simulink model "clk_tree_2"  (Simulink 7.0)
settings: Solver=ode45  StartTime=0.0  StopTime=40e-6  MaxStep=0.1e-9  RelTol=1e-3
InitFcn:
  | bit_rate=400e6;
libraries: powerlib x35, simulink x6, dspsigops x4, dspstat3 x2, commrandsrc2 x1, dspbuff3 x1, dspsnks4 x1
settings Model: Creator=dbenson  LastModifiedBy=dbenson
settings OptimizationCC: InlineInvariantSignals=on
settings DebuggingCC: SaveWithParameterizedLinksMsg=none  SignalResolutionControl=TryResolveAllWithWarning  MultiTaskDSMMsg=warning  MultiTaskCondExecSysMsg=none  StrictBusMsg=None
settings RTWCC: IncludeERTFirstTime=on
settings GRTTargetCC: TargetFcnLib=ansi_tfl_tmw.mat

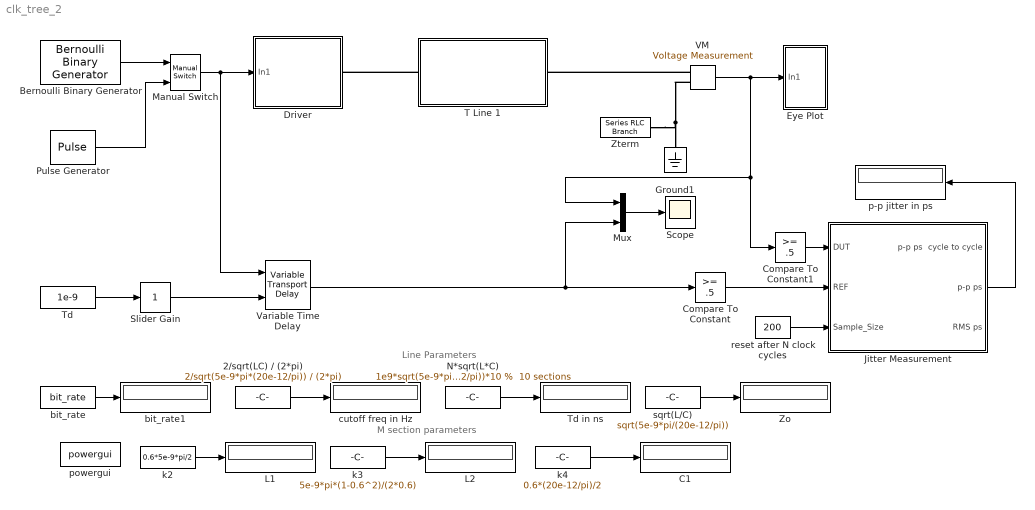
== system clk_tree_2 ==
  note: Line Parameters
  note: M section parameters
  2/sqrt(LC) / (2*pi) : Constant  Value=2/sqrt(5e-9*pi*(20e-12/pi)) / (2*pi)  OutDataType=sfix(16)  OutScaling=2^0
  Bernoulli Binary Generator : commrandsrc2/Bernoulli Binary Generator  DialogController=commDDGCreate  DialogControllerArgs=DataTag0  SystemSampleTime=-1  P=0.5  seed=61  Ts=1/bit_rate  frameBased=off  sampPerFrame=1  orient=off  outDataType=double
  C1 : Display
  Compare To Constant : simulink/Logic and Bit Operations/Compare To Constant  SystemSampleTime=-1  relop=>=  const=.5  LogicOutDataTypeMode=boolean  ZeroCross=off
  Compare To Constant1 : simulink/Logic and Bit Operations/Compare To Constant  SystemSampleTime=-1  relop=>=  const=.5  LogicOutDataTypeMode=boolean  ZeroCross=off
  Driver : Subsystem
  Eye Plot : Subsystem
  Ground1 : powerlib/Elements/Ground  Orientation=down  DialogController=POWERSYS.PowerSysDialog  PhysicalDomain=powersysdomain  SubClassName=unknown  LeftPortType=p1  RightPortType=p1  LConnTagsString=a
  "Jitter Measurement " : Subsystem
  L1 : Display
  L2 : Display
  Manual Switch : simulink/Signal Routing/Manual Switch  SystemSampleTime=-1  sw=1  action=0  varsize=off
  Mux : Mux  Inputs=2
  N*sqrt(L*C) : Constant  Value="1e9*sqrt(5e-9*pi*(20e-12/pi))*10 %  10 sections"  OutDataType=sfix(16)  OutScaling=2^0
  Pulse Generator : DiscretePulseGenerator  PulseType=Time based  Period=2/bit_rate  PulseWidth=50
  Scope : Scope
      settings: TimeRange=1e-008  YMin=-0.4162746057435363  YMax=1.209680454665211
  Slider Gain : simulink/Math Operations/Slider Gain  SystemSampleTime=-1  low=0  gain=1  high=5
  T Line 1 : Subsystem
  Td : Constant  Value=1e-9  OutDataType=sfix(16)  OutScaling=2^0
  Td in ns : Display
  VM : powerlib/Measurements/Voltage Measurement  DialogController=POWERSYS.PowerSysDialog  SystemSampleTime=-1  PhasorSimulation=off  OutputType=Complex  PSBequivalent=0
  Variable Time Delay : VariableTransportDelay  MaximumDelay=10e-9
  Zo : Display
  Zterm : powerlib/Elements/Series RLC Branch  DialogController=POWERSYS.PowerSysDialog  PhysicalDomain=powersysdomain  SubClassName=unknown  LeftPortType=p1  RightPortType=p1  LConnTagsString=__new0  RConnTagsString=__new0  BranchType=R  Resistance=50  Inductance=1e-3  SetiL0=off  InitialCurrent=0  Capacitance=1e-6  Setx0=off  InitialVoltage=0  Measurements=None
  bit_rate : Constant  Value=bit_rate  OutDataType=sfix(16)  OutScaling=2^0
  bit_rate1 : Display
  cutoff freq in Hz : Display
  k2 : Constant  Value=0.6*5e-9*pi/2  OutDataType=sfix(16)  OutScaling=2^0
  k3 : Constant  Value=5e-9*pi*(1-0.6^2)/(2*0.6)  OutDataType=sfix(16)  OutScaling=2^0
  k4 : Constant  Value=0.6*(20e-12/pi)/2  OutDataType=sfix(16)  OutScaling=2^0
  p-p jitter in ps : Display
  powergui : powerlib/powergui  SystemSampleTime=-1  SimulationMode=Continuous  SampleTime=50e-6  echomessages=off  RestoreLinks=warning  x0status=blocks  Frange=[0:2:500]  Ylog=off  Xlog=on  ShowGrid=off  save=off  variable=ZData  ZoomFFT=on  StartTime=0.0  cycles=1  DisplayStyle=1  fundamental=60  FreqAxis=off  MaxFrequency=1000  frequencyindice=0  frequencyindicesteady=1  RmsSteady=1  display=off  Ts=0  frequency=60  methode=off  HookPort=off  Interpol=off  SPID=off  FunctionMessages=off
  reset after N clock cycles : Constant  Value=200  VectorParams1D=off  OutDataType=sfix(16)  OutScaling=2^0
  sqrt(L/C) : Constant  Value=sqrt(5e-9*pi/(20e-12/pi))  OutDataType=sfix(16)  OutScaling=2^0
  wires:
  sqrt(L/C)/1 -> Zo/1
  N*sqrt(L*C)/1 -> Td in ns/1
  k2/1 -> L1/1
  k3/1 -> L2/1
  k4/1 -> C1/1
  2/sqrt(LC) / (2*pi)/1 -> cutoff freq in Hz/1
  VM/1 -> Eye Plot/1(In1), Mux/1, Compare To Constant1/1
  bit_rate/1 -> bit_rate1/1
  Pulse Generator/1 -> Manual Switch/2
  Bernoulli Binary Generator/1 -> Manual Switch/1
  Manual Switch/1 -> Driver/1(In1), Variable Time Delay/1
  "Jitter Measurement "/2(p-p ps) -> p-p jitter in ps/1
  reset after N clock cycles/1 -> "Jitter Measurement "/3(Sample_Size)
  Variable Time Delay/1 -> Mux/2, Compare To Constant/1
  Td/1 -> Slider Gain/1
  Mux/1 -> Scope/1
  Slider Gain/1 -> Variable Time Delay/2
  Compare To Constant/1 -> "Jitter Measurement "/2(REF)
  Compare To Constant1/1 -> "Jitter Measurement "/1(DUT)
  connections:
  T Line 1/LConn1 -- Driver/RConn1
  VM/LConn2 -- Ground1/LConn1 -- Zterm/RConn1
  VM/LConn1 -- T Line 1/RConn1

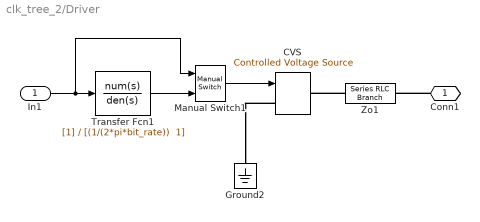
== system clk_tree_2/Driver ==
  In1 : Inport
  CVS : powerlib/Electrical Sources/Controlled Voltage Source  Description=source block  DialogController=POWERSYS.PowerSysDialog  SystemSampleTime=-1  Initialize=off  Source_Type=AC  Amplitude=0  Phase=0  Frequency=0  Measurements=None
      settings: AttributesFormatString=\n
  Ground2 : powerlib/Elements/Ground  Orientation=down  DialogController=POWERSYS.PowerSysDialog  PhysicalDomain=powersysdomain  SubClassName=unknown  LeftPortType=p1  RightPortType=p1  LConnTagsString=a
  Manual Switch1 : simulink/Signal Routing/Manual Switch  SystemSampleTime=-1  sw=0  action=0  varsize=off
  Transfer Fcn1 : TransferFcn  Denominator="[(1/(2*pi*bit_rate))  1]"
  Zo1 : powerlib/Elements/Series RLC Branch  DialogController=POWERSYS.PowerSysDialog  PhysicalDomain=powersysdomain  SubClassName=unknown  LeftPortType=p1  RightPortType=p1  LConnTagsString=__new0  RConnTagsString=__new0  BranchType=R  Resistance=50  Inductance=1e-3  SetiL0=off  InitialCurrent=0  Capacitance=1e-6  Setx0=off  InitialVoltage=0  Measurements=None
  Conn1 : PMIOPort  Orientation=left  Port=1  Side=Right
  wires:
  In1/1 -> Manual Switch1/1, Transfer Fcn1/1
  Manual Switch1/1 -> CVS/1
  Transfer Fcn1/1 -> Manual Switch1/2
  connections:
  CVS/LConn1 -- Ground2/LConn1
  Zo1/LConn1 -- CVS/RConn1
  Conn1/RConn1 -- Zo1/RConn1

== system clk_tree_2/Eye Plot ==
  In1 : Inport
  Buffer : dspbuff3/Buffer  N=200  V=0  ic=0
  Vector Scope1 : dspsnks4/Vector Scope  DialogController=dspdialog.VectorScope  DialogControllerArgs=DataTag1  ScopeProperties=on  Domain=User-defined  HorizSpan=1  DisplayProperties=off  AxisGrid=on  Memory=on  FrameNumber=on  AxisLegend=off  AxisZoom=off  OpenScopeAtSimStart=on  OpenScopeImmediately=off  FigPos=[3 39 417 270]  AxisProperties=off  XUnits=Hertz  XRange=[0...Fs/2]  InheritXIncr=off  XIncr=.01/bit_rate  XLabel=Time  XLimit=Auto  XMin=0  XMax=1  XStart=0  YUnits=dB  YLabel=Amplitude  LineProperties=off  LineColors=[0 0 1]|[1 0 0]
      settings: YMin=-0.298875449569035  YMax=1.30250670189524
  Zero-Order Hold1 : ZeroOrderHold  SampleTime=.01/bit_rate
  wires:
  Zero-Order Hold1/1 -> Buffer/1  "Clock"
  Buffer/1 -> Vector Scope1/1
  In1/1 -> Zero-Order Hold1/1

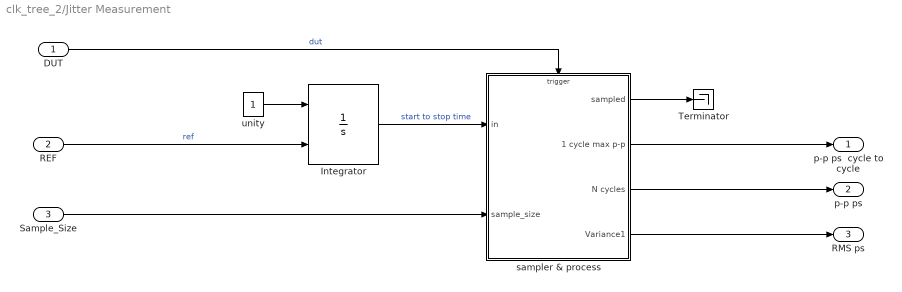
== system clk_tree_2/Jitter Measurement  ==
  DUT : Inport  OutDataType=sfix(16)  OutScaling=2^0
  REF : Inport  Port=2  OutDataType=sfix(16)  OutScaling=2^0
  Sample_Size : Inport  Port=3  OutDataType=sfix(16)  OutScaling=2^0
  Integrator : Integrator  ExternalReset=rising
  Terminator : Terminator
  sampler & process : Subsystem  TreatAsAtomicUnit=on
  unity : Constant  OutDataTypeMode=double  OutDataType=sfix(16)  OutScaling=2^0
  p-p ps  cycle to cycle : Outport  OutDataType=sfix(16)  OutScaling=2^0
  p-p ps : Outport  Port=2  OutDataType=sfix(16)  OutScaling=2^0
  RMS ps : Outport  Port=3  OutDataType=sfix(16)  OutScaling=2^0
  wires:
  DUT/1 -> sampler & process/Trigger  "dut"
  REF/1 -> Integrator/2  "ref"
  Integrator/1 -> sampler & process/1(in)  "start to stop time"
  Sample_Size/1 -> sampler & process/2(sample_size)
  sampler & process/3(N cycles) -> p-p ps/1
  sampler & process/4(Variance1) -> RMS ps/1
  unity/1 -> Integrator/1
  sampler & process/2(1 cycle max p-p) -> p-p ps  cycle to cycle/1
  sampler & process/1(sampled) -> Terminator/1

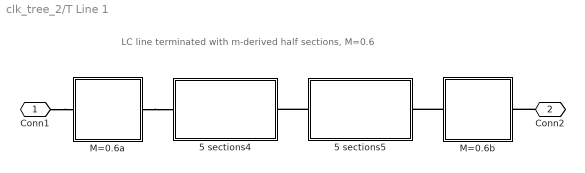
== system clk_tree_2/T Line 1 ==
  note: LC line terminated with m-derived half sections, M=0.6
  5 sections4 : Subsystem
  5 sections5 : Subsystem
  M=0.6a : Subsystem
  M=0.6b : Subsystem
  Conn1 : PMIOPort  Port=1  Side=Left
  Conn2 : PMIOPort  Orientation=left  Port=2  Side=Right
  connections:
  M=0.6a/RConn1 -- 5 sections4/LConn1
  5 sections5/LConn1 -- 5 sections4/RConn1
  M=0.6b/LConn1 -- 5 sections5/RConn1
  Conn1/RConn1 -- M=0.6a/LConn1
  Conn2/RConn1 -- M=0.6b/RConn1

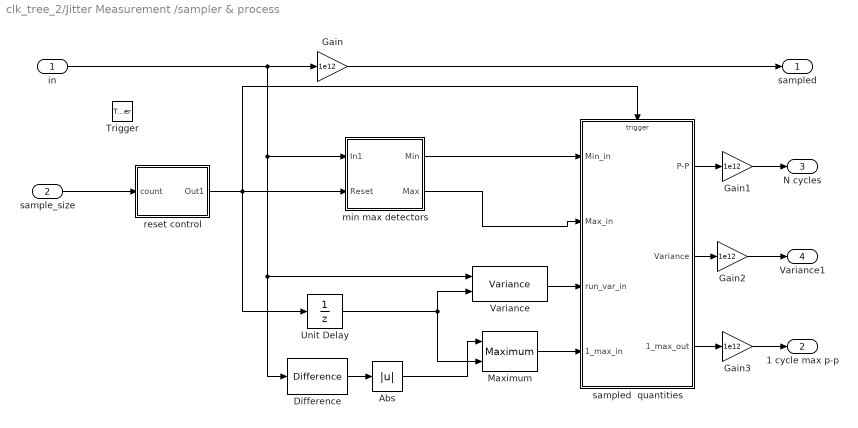
== system clk_tree_2/Jitter Measurement /sampler & process ==
  in : Inport  OutDataType=sfix(16)  OutScaling=2^0
  sample_size : Inport  Port=2  OutDataType=sfix(16)  OutScaling=2^0
  Trigger : TriggerPort
  Abs : Abs
  Difference : simulink/Discrete/Difference  SystemSampleTime=-1  ICPrevInput=0.0  OutMin=[]  OutMax=[]  OutDataType=sfix(16)  OutScaling=2^-10  DoSatur=off
  Gain{,1..3} (4 alike) : Gain  Gain=1e12  ParameterDataType=sfix(16)  ParameterScaling=2^0  OutDataType=sfix(16)  OutScaling=2^0
  Maximum : dspstat3/Maximum  DialogController=dspfixptddg.MinMax  DialogControllerArgs=DataTag2  fcn=Running  reset=Rising edge  indexBase=One  operateOver=Each column  Dimension=1  colComp=on  operation=maximum  roundingMode=Floor  overflowMode=off
  Unit Delay : UnitDelay  SampleTime=-1
  Variance : dspstat3/Variance  DialogController=dspDDGCreate  DialogControllerArgs=DataTag3  run=on  reset_popup=Rising edge  roundingMode=Floor  overflowMode=off
  min max detectors : Subsystem
  reset control : Subsystem
  sampled  quantities : Subsystem  TreatAsAtomicUnit=on
  sampled : Outport  OutDataType=sfix(16)  OutScaling=2^0
  1 cycle max p-p : Outport  Port=2  OutDataType=sfix(16)  OutScaling=2^0
  N cycles : Outport  Port=3  OutDataType=sfix(16)  OutScaling=2^0
  Variance1 : Outport  Port=4  OutDataType=sfix(16)  OutScaling=2^0
  wires:
  in/1 -> Gain/1, Variance/1, Difference/1, min max detectors/1(In1)
  Difference/1 -> Abs/1
  Abs/1 -> Maximum/1
  sample_size/1 -> reset control/1(count)
  reset control/1(Out1) -> Unit Delay/1, sampled  quantities/Trigger, min max detectors/2(Reset)
  sampled  quantities/1(P-P) -> Gain1/1
  Variance/1 -> sampled  quantities/3(run_var_in)
  sampled  quantities/2(Variance) -> Gain2/1
  Unit Delay/1 -> Variance/2, Maximum/2
  Maximum/1 -> sampled  quantities/4(1_max_in)
  sampled  quantities/3(1_max_out) -> Gain3/1
  Gain/1 -> sampled/1
  Gain1/1 -> N cycles/1
  Gain2/1 -> Variance1/1
  Gain3/1 -> 1 cycle max p-p/1
  min max detectors/2(Max) -> sampled  quantities/2(Max_in)
  min max detectors/1(Min) -> sampled  quantities/1(Min_in)

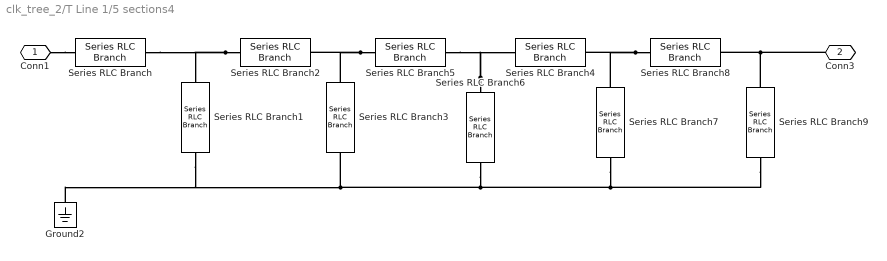
== system clk_tree_2/T Line 1/5 sections4 ==
  Ground2 : powerlib/Elements/Ground  Orientation=down  DialogController=POWERSYS.PowerSysDialog  PhysicalDomain=powersysdomain  SubClassName=unknown  LeftPortType=p1  RightPortType=p1  LConnTagsString=a
  Series RLC Branch{,2,4..5,8} (5 alike) : powerlib/Elements/Series RLC Branch  DialogController=POWERSYS.PowerSysDialog  PhysicalDomain=powersysdomain  SubClassName=unknown  LeftPortType=p1  RightPortType=p1  LConnTagsString=__new0  RConnTagsString=__new0  BranchType=L  Resistance=1.0  Inductance=5*pi*1e-9  SetiL0=off  InitialCurrent=0  Capacitance=1.0  Setx0=off  InitialVoltage=0  Measurements=None
  Series RLC Branch{1,3,6..7,9} (5 alike) : powerlib/Elements/Series RLC Branch  Orientation=down  DialogController=POWERSYS.PowerSysDialog  PhysicalDomain=powersysdomain  SubClassName=unknown  LeftPortType=p1  RightPortType=p1  LConnTagsString=__new0  RConnTagsString=__new0  BranchType=C  Resistance=1.0  Inductance=1.0  SetiL0=off  InitialCurrent=0  Capacitance=20e-12/pi  Setx0=off  InitialVoltage=0  Measurements=None
  Conn1 : PMIOPort  Port=1  Side=Left
  Conn3 : PMIOPort  Orientation=left  Port=2  Side=Right
  connections:
  Conn1/RConn1 -- Series RLC Branch/LConn1
  Conn3/RConn1 -- Series RLC Branch8/RConn1 -- Series RLC Branch9/LConn1
  Series RLC Branch8/LConn1 -- Series RLC Branch4/RConn1 -- Series RLC Branch7/LConn1
  Series RLC Branch6/LConn1 -- Series RLC Branch4/LConn1 -- Series RLC Branch5/RConn1
  Series RLC Branch5/LConn1 -- Series RLC Branch2/RConn1 -- Series RLC Branch3/LConn1
  Series RLC Branch9/RConn1 -- Series RLC Branch7/RConn1 -- Series RLC Branch1/RConn1 -- Ground2/LConn1 -- Series RLC Branch3/RConn1 -- Series RLC Branch6/RConn1
  Series RLC Branch2/LConn1 -- Series RLC Branch1/LConn1 -- Series RLC Branch/RConn1

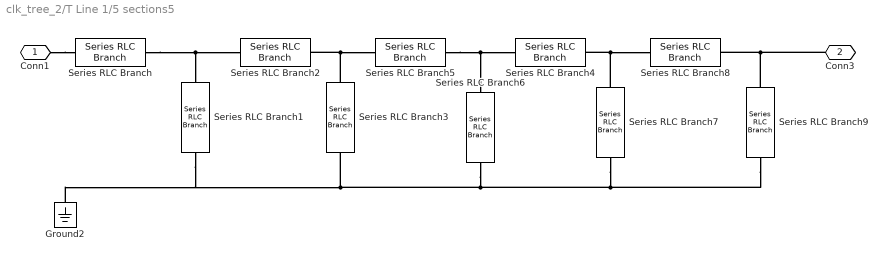
== system clk_tree_2/T Line 1/5 sections5 ==
  Ground2 : powerlib/Elements/Ground  Orientation=down  DialogController=POWERSYS.PowerSysDialog  PhysicalDomain=powersysdomain  SubClassName=unknown  LeftPortType=p1  RightPortType=p1  LConnTagsString=a
  Series RLC Branch{,2,4..5,8} (5 alike) : powerlib/Elements/Series RLC Branch  DialogController=POWERSYS.PowerSysDialog  PhysicalDomain=powersysdomain  SubClassName=unknown  LeftPortType=p1  RightPortType=p1  LConnTagsString=__new0  RConnTagsString=__new0  BranchType=L  Resistance=1.0  Inductance=5*pi*1e-9  SetiL0=off  InitialCurrent=0  Capacitance=1.0  Setx0=off  InitialVoltage=0  Measurements=None
  Series RLC Branch{1,3,6..7,9} (5 alike) : powerlib/Elements/Series RLC Branch  Orientation=down  DialogController=POWERSYS.PowerSysDialog  PhysicalDomain=powersysdomain  SubClassName=unknown  LeftPortType=p1  RightPortType=p1  LConnTagsString=__new0  RConnTagsString=__new0  BranchType=C  Resistance=1.0  Inductance=1.0  SetiL0=off  InitialCurrent=0  Capacitance=20e-12/pi  Setx0=off  InitialVoltage=0  Measurements=None
  Conn1 : PMIOPort  Port=1  Side=Left
  Conn3 : PMIOPort  Orientation=left  Port=2  Side=Right
  connections:
  Series RLC Branch/RConn1 -- Series RLC Branch1/LConn1 -- Series RLC Branch2/LConn1
  Series RLC Branch9/RConn1 -- Series RLC Branch6/RConn1 -- Series RLC Branch3/RConn1 -- Series RLC Branch1/RConn1 -- Ground2/LConn1 -- Series RLC Branch7/RConn1
  Series RLC Branch3/LConn1 -- Series RLC Branch2/RConn1 -- Series RLC Branch5/LConn1
  Series RLC Branch5/RConn1 -- Series RLC Branch4/LConn1 -- Series RLC Branch6/LConn1
  Series RLC Branch7/LConn1 -- Series RLC Branch4/RConn1 -- Series RLC Branch8/LConn1
  Series RLC Branch9/LConn1 -- Series RLC Branch8/RConn1 -- Conn3/RConn1
  Conn1/RConn1 -- Series RLC Branch/LConn1

== system clk_tree_2/T Line 1/M=0.6a ==
  Ground2 : powerlib/Elements/Ground  Orientation=down  DialogController=POWERSYS.PowerSysDialog  PhysicalDomain=powersysdomain  SubClassName=unknown  LeftPortType=p1  RightPortType=p1  LConnTagsString=a
  Series RLC Branch : powerlib/Elements/Series RLC Branch  DialogController=POWERSYS.PowerSysDialog  PhysicalDomain=powersysdomain  SubClassName=unknown  LeftPortType=p1  RightPortType=p1  LConnTagsString=__new0  RConnTagsString=__new0  BranchType=L  Resistance=1.0  Inductance=4.712e-9  SetiL0=off  InitialCurrent=0  Capacitance=1.0  Setx0=off  InitialVoltage=0  Measurements=None
  rlc : powerlib/Elements/Series RLC Branch  Orientation=down  DialogController=POWERSYS.PowerSysDialog  PhysicalDomain=powersysdomain  SubClassName=unknown  LeftPortType=p1  RightPortType=p1  LConnTagsString=__new0  RConnTagsString=__new0  BranchType=LC  Resistance=1.0  Inductance=8.378e-9  SetiL0=off  InitialCurrent=0  Capacitance=1.91e-12  Setx0=off  InitialVoltage=0  Measurements=None
  C1 : PMIOPort  Port=1  Side=Left
  C3 : PMIOPort  Orientation=left  Port=2  Side=Right
  connections:
  C3/RConn1 -- rlc/LConn1 -- Series RLC Branch/RConn1
  C1/RConn1 -- Series RLC Branch/LConn1
  Ground2/LConn1 -- rlc/RConn1

== system clk_tree_2/T Line 1/M=0.6b ==
  Ground2 : powerlib/Elements/Ground  Orientation=down  DialogController=POWERSYS.PowerSysDialog  PhysicalDomain=powersysdomain  SubClassName=unknown  LeftPortType=p1  RightPortType=p1  LConnTagsString=a
  Series RLC Branch : powerlib/Elements/Series RLC Branch  DialogController=POWERSYS.PowerSysDialog  PhysicalDomain=powersysdomain  SubClassName=unknown  LeftPortType=p1  RightPortType=p1  LConnTagsString=__new0  RConnTagsString=__new0  BranchType=L  Resistance=1.0  Inductance=4.712e-9  SetiL0=off  InitialCurrent=0  Capacitance=1.0  Setx0=off  InitialVoltage=0  Measurements=None
  rlc : powerlib/Elements/Series RLC Branch  Orientation=down  DialogController=POWERSYS.PowerSysDialog  PhysicalDomain=powersysdomain  SubClassName=unknown  LeftPortType=p1  RightPortType=p1  LConnTagsString=__new0  RConnTagsString=__new0  BranchType=LC  Resistance=1.0  Inductance=8.378e-9  SetiL0=off  InitialCurrent=0  Capacitance=1.91e-12  Setx0=off  InitialVoltage=0  Measurements=None
  C1 : PMIOPort  Port=1  Side=Left
  C3 : PMIOPort  Orientation=left  Port=2  Side=Right
  connections:
  C1/RConn1 -- Series RLC Branch/LConn1
  Ground2/LConn1 -- rlc/RConn1
  Series RLC Branch/RConn1 -- rlc/LConn1 -- C3/RConn1

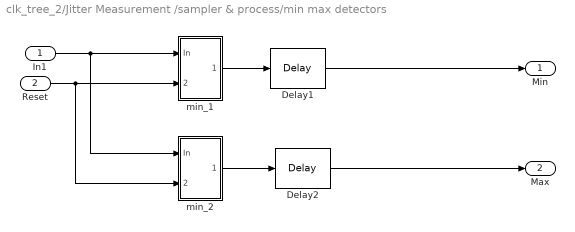
== system clk_tree_2/Jitter Measurement /sampler & process/min max detectors ==
  In1 : Inport  OutDataType=sfix(16)  OutScaling=2^0
  Reset : Inport  Port=2  OutDataType=sfix(16)  OutScaling=2^0
  Delay1 : dspsigops/Delay  dly_unit=Samples  delay=1  ic_detail=off  dif_ic_for_ch=off  dif_ic_for_dly=off  ic=0  reset_popup=None
  Delay2 : dspsigops/Delay  dly_unit=Samples  delay=1  ic_detail=off  dif_ic_for_ch=off  dif_ic_for_dly=off  ic=0  reset_popup=None
  min_1 : Subsystem
  min_2 : Subsystem
  Min : Outport  OutDataType=sfix(16)  OutScaling=2^0
  Max : Outport  Port=2  OutDataType=sfix(16)  OutScaling=2^0
  wires:
  Reset/1 -> min_1/2(Rst), min_2/2(Rst)
  In1/1 -> min_1/1(In), min_2/1(In)
  min_1/1(Out) -> Delay1/1
  min_2/1(Out) -> Delay2/1
  Delay1/1 -> Min/1
  Delay2/1 -> Max/1

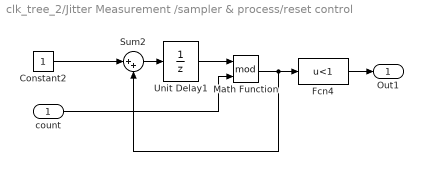
== system clk_tree_2/Jitter Measurement /sampler & process/reset control ==
  count : Inport  OutDataType=sfix(16)  OutScaling=2^0
  Constant2 : Constant  OutDataType=sfix(16)  OutScaling=2^0
  Fcn4 : Fcn  Expr=u<1
  Math Function : Math  Operator=mod  OutDataType=sfix(16)  OutScaling=2^0  SaturateOnIntegerOverflow=on
  Sum2 : Sum  Inputs=|++  OutDataType=sfix(16)  OutScaling=2^0  SaturateOnIntegerOverflow=on  InputSameDT=on
  Unit Delay1 : UnitDelay  SampleTime=-1
  Out1 : Outport  OutDataType=sfix(16)  OutScaling=2^0
  wires:
  Math Function/1 -> Fcn4/1, Sum2/2
  Unit Delay1/1 -> Math Function/1
  Constant2/1 -> Sum2/1
  Sum2/1 -> Unit Delay1/1
  Fcn4/1 -> Out1/1
  count/1 -> Math Function/2

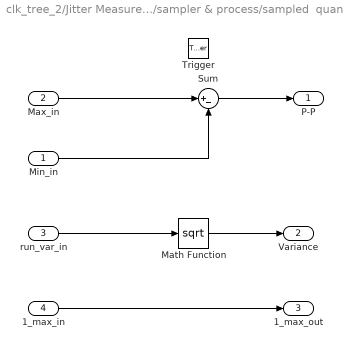
== system clk_tree_2/Jitter Measurement /sampler & process/sampled  quantities ==
  Min_in : Inport  OutDataType=sfix(16)  OutScaling=2^0
  Max_in : Inport  Port=2  OutDataType=sfix(16)  OutScaling=2^0
  run_var_in : Inport  Port=3  OutDataType=sfix(16)  OutScaling=2^0
  1_max_in : Inport  Port=4  OutDataType=sfix(16)  OutScaling=2^0
  Trigger : TriggerPort
  Math Function : Math  Operator=sqrt  OutDataType=sfix(16)  OutScaling=2^0  SaturateOnIntegerOverflow=on
  Sum : Sum  Inputs=|+-  OutDataType=sfix(16)  OutScaling=2^0  SaturateOnIntegerOverflow=on  InputSameDT=on
  P-P : Outport  OutDataType=sfix(16)  OutScaling=2^0
  Variance : Outport  Port=2  OutDataType=sfix(16)  OutScaling=2^0
  1_max_out : Outport  Port=3  OutDataType=sfix(16)  OutScaling=2^0
  wires:
  Max_in/1 -> Sum/1
  Min_in/1 -> Sum/2
  Sum/1 -> P-P/1
  Math Function/1 -> Variance/1
  run_var_in/1 -> Math Function/1
  1_max_in/1 -> 1_max_out/1

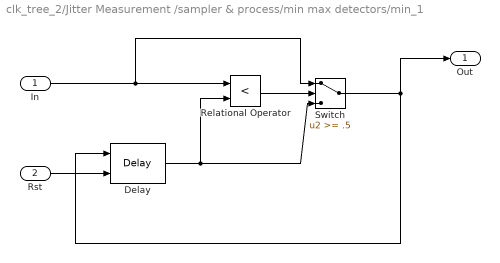
== system clk_tree_2/Jitter Measurement /sampler & process/min max detectors/min_1 ==
  In : Inport  OutDataType=sfix(16)  OutScaling=2^0
  Rst : Inport  Port=2  OutDataType=sfix(16)  OutScaling=2^0
  Delay : dspsigops/Delay  dly_unit=Samples  delay=1  ic_detail=off  dif_ic_for_ch=off  dif_ic_for_dly=off  ic=1e6  reset_popup=Non-zero sample
  Relational Operator : RelationalOperator  Operator=<  LogicOutDataTypeMode=boolean
  Switch : Switch  Threshold=.5
  Out : Outport  OutDataType=sfix(16)  OutScaling=2^0
  wires:
  In/1 -> Relational Operator/1, Switch/1
  Rst/1 -> Delay/2
  Delay/1 -> Relational Operator/2, Switch/3
  Relational Operator/1 -> Switch/2
  Switch/1 -> Delay/1, Out/1

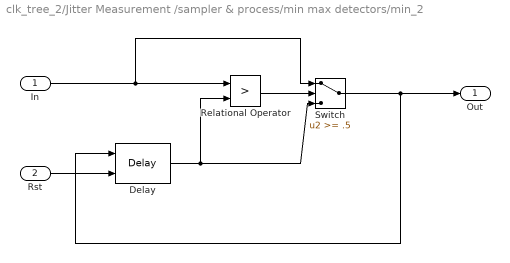
== system clk_tree_2/Jitter Measurement /sampler & process/min max detectors/min_2 ==
  In : Inport  OutDataType=sfix(16)  OutScaling=2^0
  Rst : Inport  Port=2  OutDataType=sfix(16)  OutScaling=2^0
  Delay : dspsigops/Delay  dly_unit=Samples  delay=1  ic_detail=off  dif_ic_for_ch=off  dif_ic_for_dly=off  ic=-1e6  reset_popup=Non-zero sample
  Relational Operator : RelationalOperator  Operator=>  LogicOutDataTypeMode=boolean
  Switch : Switch  Threshold=.5
  Out : Outport  OutDataType=sfix(16)  OutScaling=2^0
  wires:
  Switch/1 -> Out/1, Delay/1
  Relational Operator/1 -> Switch/2
  Delay/1 -> Switch/3, Relational Operator/2
  Rst/1 -> Delay/2
  In/1 -> Switch/1, Relational Operator/1
